simulink model "myModel_observer"  (R2023b)
settings: Solver=VariableStepAuto  StartTime=0.0  StopTime=10  RelTol=1e-3
values from neighbouring files (symbols this model uses):
  A = [0, 0               ,   1           , 0 ... (first row only)    [mytask.m]
  Ad = sys_d.a    [mytask.m]
  B = [0, 0,  1/mc,   1/(L*mc)]'    [mytask.m]
  Bd = sys_d.b    [mytask.m]
  C = [1, 0,  0,  0]    [mytask.m]
  Cd = sys_d.c    [mytask.m]
  K_d = acker(Ad,Bd,des_poles_d)    [mytask.m]
  Ob = acker(Ad',Cd',des_poles_Ob)    [mytask.m]
  Ts = 0.1    [mytask.m]
  x0 = [0;    5*pi/180;   0;  0]    [mytask.m]
settings Model: Creator=admin  LastModifiedBy=admin

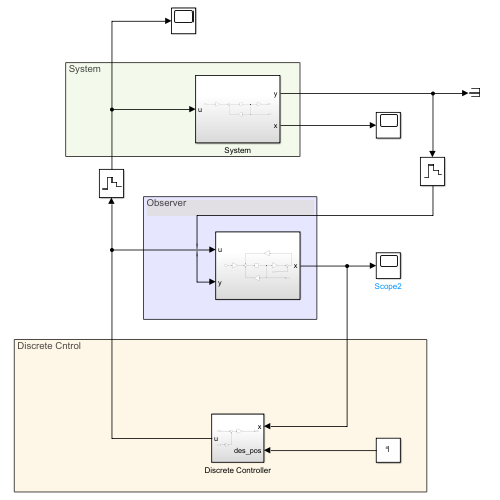
[thumbnail: Simulink's stored preview of the top-level diagram]
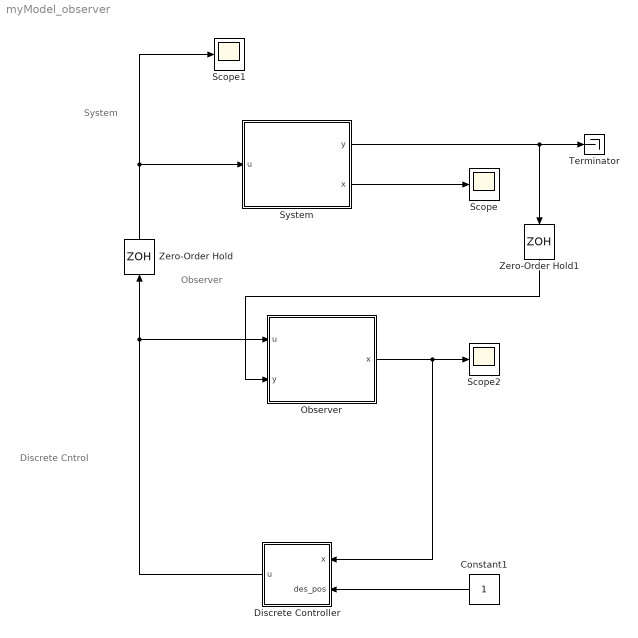
== system myModel_observer ==
  note: Observer
  note: System
  note: Discrete Cntrol
  Constant1 : Constant
  Discrete Controller : Subsystem
  Observer : Subsystem
  Scope : Scope
  Scope1 : Scope
  Scope2 : Scope
  System : Subsystem
  Terminator : Terminator
  Zero-Order Hold : ZeroOrderHold  SampleTime=Ts
  Zero-Order Hold1 : ZeroOrderHold  SampleTime=Ts
  wires:
  System/1(y) -> Zero-Order Hold1/1, Terminator/1
  System/2(x) -> Scope/1
  Constant1/1 -> Discrete Controller/2(des_pos)
  Discrete Controller/1(u) -> Zero-Order Hold/1, Observer/1(u)
  Zero-Order Hold/1 -> System/1(u), Scope1/1
  Zero-Order Hold1/1 -> Observer/2(y)
  Observer/1(x) -> Discrete Controller/1(x), Scope2/1

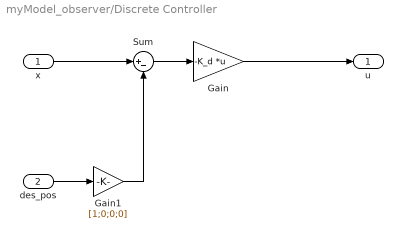
== system myModel_observer/Discrete Controller ==
  x : Inport
  des_pos : Inport  Port=2
  Gain : Gain  Gain=-K_d  Multiplication=Matrix(K*u)
  Gain1 : Gain  Gain=[1;0;0;0]
  Sum : Sum  Inputs=|+-
  u : Outport
  wires:
  Gain/1 -> u/1
  Sum/1 -> Gain/1
  x/1 -> Sum/1
  des_pos/1 -> Gain1/1
  Gain1/1 -> Sum/2

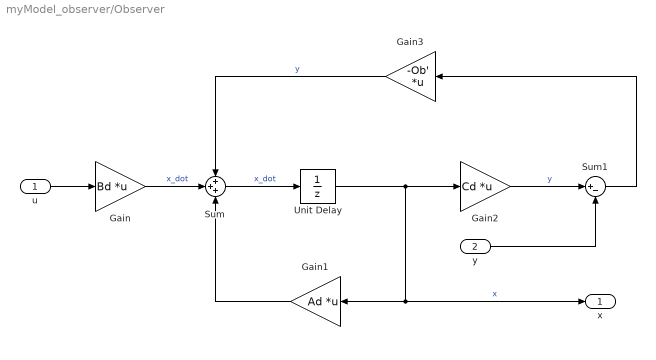
== system myModel_observer/Observer ==
  u : Inport
  y : Inport  Port=2
  Gain : Gain  Gain=Bd  Multiplication=Matrix(K*u)
  Gain1 : Gain  Gain=Ad  Multiplication=Matrix(K*u)
  Gain2 : Gain  Gain=Cd  Multiplication=Matrix(K*u)
  Gain3 : Gain  Gain=-Ob'  Multiplication=Matrix(K*u)
  Sum : Sum  Inputs=+++
  Sum1 : Sum  Inputs=|+-
  Unit Delay : UnitDelay  InitialCondition=x0*0  SampleTime=-1  HasFrameUpgradeWarning=on
  x : Outport
  wires:
  Sum/1 -> Unit Delay/1  "x_dot"
  Unit Delay/1 -> Gain2/1, x/1, Gain1/1  "x"
  u/1 -> Gain/1
  Gain/1 -> Sum/2  "x_dot"
  Gain1/1 -> Sum/3
  Gain2/1 -> Sum1/1  "y"
  y/1 -> Sum1/2
  Sum1/1 -> Gain3/1
  Gain3/1 -> Sum/1  "y"

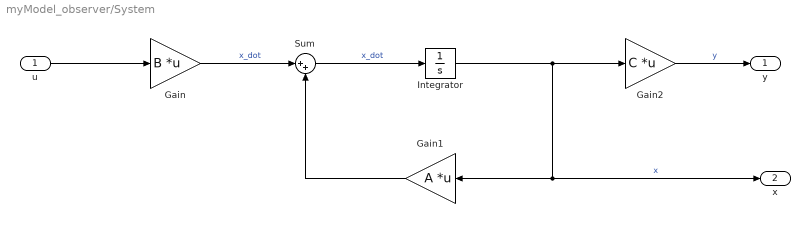
== system myModel_observer/System ==
  u : Inport
  Gain : Gain  Gain=B  Multiplication=Matrix(K*u)
  Gain1 : Gain  Gain=A  Multiplication=Matrix(K*u)
  Gain2 : Gain  Gain=C  Multiplication=Matrix(K*u)
  Integrator : Integrator  InitialCondition=x0
  Sum : Sum  Inputs=|++
  y : Outport
  x : Outport  Port=2
  wires:
  Gain/1 -> Sum/1  "x_dot"
  Gain2/1 -> y/1  "y"
  Sum/1 -> Integrator/1  "x_dot"
  Gain1/1 -> Sum/2
  Integrator/1 -> x/1, Gain1/1, Gain2/1  "x"
  u/1 -> Gain/1
